simulink model "cic2_1000"  (Simulink 6.6)
settings: Solver=FixedStepDiscrete  SolverMode=MultiTasking  StartTime=0.0  StopTime=10.0  RelTol=1e-3
libraries: dspsigops x7, dspsrcs4 x1
settings Model: Creator=svenhoffmann  LastModifiedBy=svenhoffmann  ExtModeAutoUpdateStatusClock=off
settings DebuggingCC: SignalResolutionControl=TryResolveAllWithWarning  MultiTaskDSMMsg=warning  MultiTaskCondExecSysMsg=none  StrictBusMsg=None
settings RTWCC: IncludeERTFirstTime=on

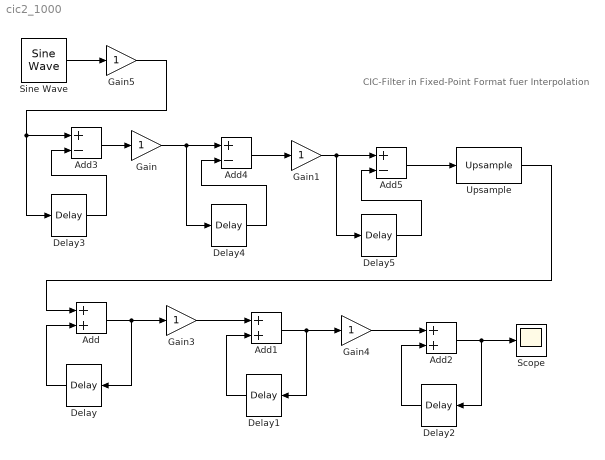
== system cic2_1000 ==
  note: CIC-Filter
      | in Fixed-Point
      | Format
      | fuer Interpolation
  Add : Sum  OutScaling=2^-15
  Add1 : Sum  OutScaling=2^-10
  Add2 : Sum  OutScaling=2^-10
  Add3 : Sum  Inputs=+-  OutScaling=2^-12
  Add4 : Sum  Inputs=+-  OutScaling=2^-10
  Add5 : Sum  Inputs=+-  OutScaling=2^-8
  Delay : dspsigops/Delay  Orientation=left  dly_unit=Samples  delay=1  ic_detail=off  dif_ic_for_ch=off  dif_ic_for_dly=off  ic=0  reset_popup=None
  Delay1 : dspsigops/Delay  Orientation=left  dly_unit=Samples  delay=1  ic_detail=off  dif_ic_for_ch=off  dif_ic_for_dly=off  ic=0  reset_popup=None
  Delay2 : dspsigops/Delay  Orientation=left  dly_unit=Samples  delay=1  ic_detail=off  dif_ic_for_ch=off  dif_ic_for_dly=off  ic=0  reset_popup=None
  Delay3 : dspsigops/Delay  dly_unit=Samples  delay=1  ic_detail=off  dif_ic_for_ch=off  dif_ic_for_dly=off  ic=0  reset_popup=None
  Delay4 : dspsigops/Delay  dly_unit=Samples  delay=1  ic_detail=off  dif_ic_for_ch=off  dif_ic_for_dly=off  ic=0  reset_popup=None
  Delay5 : dspsigops/Delay  dly_unit=Samples  delay=1  ic_detail=off  dif_ic_for_ch=off  dif_ic_for_dly=off  ic=0  reset_popup=None
  Gain : Gain  OutDataTypeMode=Specify via dialog  OutDataType=sfix(10)
  Gain1 : Gain  OutDataTypeMode=Specify via dialog  OutDataType=sfix(11)
  Gain3 : Gain  OutDataTypeMode=Specify via dialog  OutDataType=sfix(19)
  Gain4 : Gain  OutDataTypeMode=Specify via dialog  OutDataType=sfix(28)
  Gain5 : Gain  OutDataTypeMode=Specify via dialog  OutDataType=sfix(9)
  Scope : Scope
      settings: YMin=-1.5e+08  YMax=1.5e+08
  Sine Wave : dspsrcs4/Sine Wave  Amplitude=127  Frequency=0.5  Phase=0  SampleMode=Discrete  OutComplex=Real  CompMethod=Table lookup  TableSize=Speed  SampleTime=1/10  SamplesPerFrame=1  dataType=Fixed-point  wordLen=8  udDataType=sfix(16)  fracBitsMode=User-defined  numFracBits=0  ResetState=Restart at time zero
  Upsample : dspsigops/Upsample  N=1000  phase=0  ic=0  mode=Maintain input frame size
  wires:
  Delay/1 -> Add/2
  Add/1 -> Delay/1, Gain3/1
  Delay1/1 -> Add1/2
  Add1/1 -> Delay1/1, Gain4/1
  Add2/1 -> Delay2/1, Scope/1
  Delay2/1 -> Add2/2
  Delay3/1 -> Add3/2
  Delay4/1 -> Add4/2
  Delay5/1 -> Add5/2
  Add3/1 -> Gain/1
  Add4/1 -> Gain1/1
  Add5/1 -> Upsample/1
  Gain/1 -> Delay4/1, Add4/1
  Gain1/1 -> Delay5/1, Add5/1
  Upsample/1 -> Add/1
  Gain3/1 -> Add1/1
  Gain4/1 -> Add2/1
  Sine Wave/1 -> Gain5/1
  Gain5/1 -> Add3/1, Delay3/1
